simulink model "cac_ut"  (Simulink 8.1)
settings: Solver=FixedStepDiscrete  StartTime=0.0  StopTime=Inf  FixedStep=0.005  RelTol=1e-3
PostLoadFcn:
  | , if any(exist('dsrtsu_mdlpostloadfcn', 'file') == [2, 3, 6]), try dsrtsu_mdlpostloadfcn('Execute', bdroot); catch fprintf('Error in PostLoadFcn (dsrtsu_mdlpostloadfcn) for model "%s":\n %s\n', bdroot, lasterr); end, end,
libraries: siltestlib x29, cac x1
settings Model: DSRTSU_INTERNAL_RTI_VER=450  DSRTSU_INTERNAL_RTI_TYPE=rti1401  RTICANMMDATA=struct('GeneralSetupData',struct('modelroot','D:\ELN150201_TAIWAN\trunk\AdasDragon\software\sw_development\arch\app\acc','generalsettings',struct('filesettings',struct('destfolder',struct('Name','RTICANMM_FILES','Check',1),'buildfolder',struct('Name','.','Check',1),'AbsDestfolder',struct('Name','D:\ELN150201_TAIWAN\trunk\AdasDragon\software\sw_development\arch\app\acc\RTICANMM_FILES'),'AbsBuildfolder',struct('Name','D:\ELN150201_TAIWAN\trunk\AdasDragon\software\sw_development\arch\app\acc'))),'options',struct('addpaths',1,'rmpaths',1,'addtrcexclusion',logical(1),'cannavigator',struct('checkmonitoring',0),'show_usrtrc',0,'use_usrtrc',0),'advanced',struct('options',[1 1 1 1 1 1 1 1 1 1 1 1 1 1 1 1 1 1 1 1 1 1 1 1 1 1 1 1 1 1 1 1 1 1 1 1 1 1 1 1 1 1 1 1 1 1 1 1 1 1 1 1 1 1 1 1 1 1 1 1 1 1 1 1 1 1 1 1 1 1 1 1 1 1 1 1 1 1 1 1 1 1 1 1 1 1 1 1 1 1 1 1 1 1 1 1 1 1 1 1]),'MPSetup',{{}},'modelname','cac_ut','block','cac_ut'))  DSRTSU_INTERNAL_RTIFPGA=40  Creator=AT015411  LastModifiedBy=AT015555  BufferReuse=off
settings DataIOCC: SignalLoggingSaveFormat=Dataset
settings OptimizationCC: BlockReduction=off  OptimizeBlockIOStorage=off  BufferReuse=off  ExpressionFolding=off  ExpressionDepthLimit=128  LocalBlockOutputs=off
settings DebuggingCC: FcnCallInpInsideContextMsg=EnableAllAsError
settings HardwareCC: ProdIntDivRoundTo=Zero  ProdEndianess=BigEndian  ProdHWDeviceType=Generic->Custom  TargetIntDivRoundTo=Zero  TargetEndianess=BigEndian  TargetHWDeviceType=Generic->Custom
settings RTWCC: SystemTargetFile=rti1005.tlc  MakeCommand=make_rti  TemplateMakefile=rti1005.tmf  Description=dSPACE DS1005 Hardware Platform  ProcessScript=rti1005_make_rtw_hook
settings STFCustomTargetCC: CodeReplacementLibrary=ANSI_C  ParMdlRefBuildCompliant=on  GeneratePreprocessorConditionals=Disable all  MatFileLogging=on  SystemTargetFile=rti1005.tlc
settings GRTTargetCC: CompOptLevelCompliant=off  ConcurrentExecutionCompliant=off  ExtModeMexFile=noextcomm
settings CustomProperty: DataType=RTWOptions_EnumType_C__Program Files (x86)_dSPACE RCPHIL 2014-B_MATLAB_RTI_RTI1401_TLC_rti1005_1InitialSimState  Value=RUN
settings EnumStrPairs: String=RUN

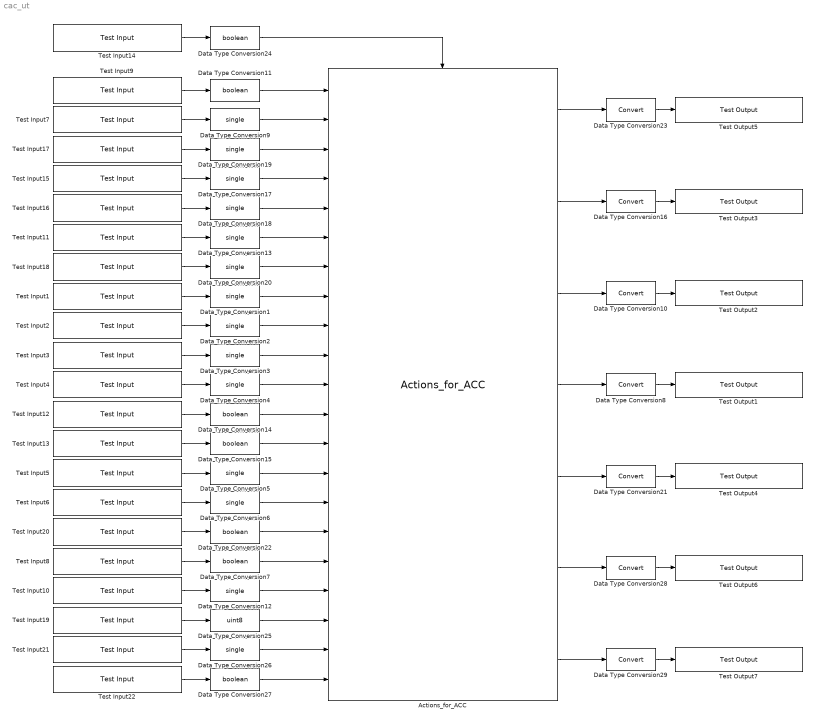
== system cac_ut ==
  Actions_for_ACC : cac/Actions_for_ACC
  Data Type Conversion{1..6,9,12..13,17..20,26} (14 alike) : DataTypeConversion  OutDataTypeStr=single
  Data Type Conversion{8,10,16,21,23,28..29} (7 alike) : DataTypeConversion
  Data Type Conversion{7,11,14..15,22,24,27} (7 alike) : DataTypeConversion  OutDataTypeStr=boolean
  Data Type Conversion25 : DataTypeConversion  OutDataTypeStr=uint8
  Test Input1 : siltestlib/Test Input  varname=VIFO_ACCTargetVehRelSpeedX_mps  sampletime=0.005
  Test Input10 : siltestlib/Test Input  varname=VJUD_VehSpd_kph  sampletime=0.005
  Test Input11 : siltestlib/Test Input  varname=VDINR_CurDriverTqReq_Nm  sampletime=0.005
  Test Input12 : siltestlib/Test Input  varname=VIFO_ACCSetSpdDec_flg  sampletime=0.005
  Test Input13 : siltestlib/Test Input  varname=VIFO_ACCResSpdInc_flg  sampletime=0.005
  Test Input14 : siltestlib/Test Input  varname=VACC_ACCActing_flg  sampletime=0.005
  Test Input15 : siltestlib/Test Input  varname=VDINR_EngTqMax_Nm  sampletime=0.005
  Test Input16 : siltestlib/Test Input  varname=VDINR_EngTqMin_Nm  sampletime=0.005
  Test Input17 : siltestlib/Test Input  varname=VDINR_LongAccel_G  sampletime=0.005
  Test Input18 : siltestlib/Test Input  varname=VDINR_LatAccel_G  sampletime=0.005
  Test Input19 : siltestlib/Test Input  varname=VACC_ACCSystemState_enum  sampletime=0.005
  Test Input2 : siltestlib/Test Input  varname=VIFO_ACCVehClearance_m  sampletime=0.005
  Test Input20 : siltestlib/Test Input  varname=VACC_ACCTargetVehAssigned_flg  sampletime=0.005
  Test Input21 : siltestlib/Test Input  varname=VJUD_VehSpd_mps  sampletime=0.005
  Test Input22 : siltestlib/Test Input  varname=VIFO_DriverTurnSignalOn_flg  sampletime=0.005
  Test Input3 : siltestlib/Test Input  varname=VJUD_ACCSetTimeGap_s  sampletime=0.005
  Test Input4 : siltestlib/Test Input  varname=VJUD_ACCSetSpeed_kph  sampletime=0.005
  Test Input5 : siltestlib/Test Input  varname=VIFO_ACCTGap_s  sampletime=0.005
  Test Input6 : siltestlib/Test Input  varname=VIFO_ACCMCLongAcc_mps2  sampletime=0.005
  Test Input7 : siltestlib/Test Input  varname=VDINR_EngTqIndicated_Nm  sampletime=0.005
  Test Input8 : siltestlib/Test Input  varname=VIFO_ACCDist_flg  sampletime=0.005
  Test Input9 : siltestlib/Test Input  varname=VACC_ACCOverride_flg  sampletime=0.005
  Test Output1 : siltestlib/Test Output  varname=VACC_ACCTorqueReq_Nm  sampletime=-1
  Test Output2 : siltestlib/Test Output  varname=VACC_ACCRawTorqueReq_Nm  sampletime=-1
  Test Output3 : siltestlib/Test Output  varname=VACC_ACCWarningReq_flg  sampletime=-1
  Test Output4 : siltestlib/Test Output  varname=VACC_ACCHoldReqEnable_flg  sampletime=-1
  Test Output5 : siltestlib/Test Output  varname=VACC_ACCDecelReq_mps2  sampletime=-1
  Test Output6 : siltestlib/Test Output  varname=VACC_ACCHoldReqDisable_flg  sampletime=-1
  Test Output7 : siltestlib/Test Output  varname=VACC_DesiredDistance_m  sampletime=-1
  wires:
  Test Input9/1 -> Data Type Conversion11/1
  Test Input10/1 -> Data Type Conversion12/1
  Test Input7/1 -> Data Type Conversion9/1
  Test Input17/1 -> Data Type Conversion19/1
  Test Input18/1 -> Data Type Conversion20/1
  Test Input15/1 -> Data Type Conversion17/1
  Test Input16/1 -> Data Type Conversion18/1
  Test Input11/1 -> Data Type Conversion13/1
  Test Input1/1 -> Data Type Conversion1/1
  Test Input2/1 -> Data Type Conversion2/1
  Test Input12/1 -> Data Type Conversion14/1
  Test Input13/1 -> Data Type Conversion15/1
  Test Input3/1 -> Data Type Conversion3/1
  Test Input4/1 -> Data Type Conversion4/1
  Test Input5/1 -> Data Type Conversion5/1
  Test Input6/1 -> Data Type Conversion6/1
  Test Input20/1 -> Data Type Conversion22/1
  Test Input8/1 -> Data Type Conversion7/1
  Data Type Conversion8/1 -> Test Output1/1
  Data Type Conversion10/1 -> Test Output2/1
  Data Type Conversion16/1 -> Test Output3/1
  Data Type Conversion21/1 -> Test Output4/1
  Data Type Conversion23/1 -> Test Output5/1
  Actions_for_ACC/1 -> Data Type Conversion23/1
  Test Input14/1 -> Data Type Conversion24/1
  Test Input19/1 -> Data Type Conversion25/1
  Test Input21/1 -> Data Type Conversion26/1
  Test Input22/1 -> Data Type Conversion27/1
  Data Type Conversion28/1 -> Test Output6/1
  Data Type Conversion29/1 -> Test Output7/1
  Actions_for_ACC/2 -> Data Type Conversion16/1
  Actions_for_ACC/3 -> Data Type Conversion10/1
  Actions_for_ACC/4 -> Data Type Conversion8/1
  Actions_for_ACC/5 -> Data Type Conversion21/1
  Actions_for_ACC/6 -> Data Type Conversion28/1
  Actions_for_ACC/7 -> Data Type Conversion29/1
  Data Type Conversion7/1 -> Actions_for_ACC/17
  Data Type Conversion3/1 -> Actions_for_ACC/10
  Data Type Conversion4/1 -> Actions_for_ACC/11
  Data Type Conversion5/1 -> Actions_for_ACC/14
  Data Type Conversion6/1 -> Actions_for_ACC/15
  Data Type Conversion9/1 -> Actions_for_ACC/2
  Data Type Conversion1/1 -> Actions_for_ACC/8
  Data Type Conversion13/1 -> Actions_for_ACC/6
  Data Type Conversion11/1 -> Actions_for_ACC/1
  Data Type Conversion12/1 -> Actions_for_ACC/18
  Data Type Conversion14/1 -> Actions_for_ACC/12
  Data Type Conversion19/1 -> Actions_for_ACC/3
  Data Type Conversion18/1 -> Actions_for_ACC/5
  Data Type Conversion22/1 -> Actions_for_ACC/16
  Data Type Conversion15/1 -> Actions_for_ACC/13
  Data Type Conversion2/1 -> Actions_for_ACC/9
  Data Type Conversion17/1 -> Actions_for_ACC/4
  Data Type Conversion20/1 -> Actions_for_ACC/7
  Data Type Conversion26/1 -> Actions_for_ACC/20
  Data Type Conversion27/1 -> Actions_for_ACC/21
  Data Type Conversion25/1 -> Actions_for_ACC/19
  Data Type Conversion24/1 -> Actions_for_ACC/Enable
